simulink model "XSWIFT_cruise"  (R2025b)
settings: Solver=ode4  StartTime=0.0  StopTime=85  FixedStep=0.001  MaxStep=0.001  RelTol=1e-4
InitFcn:
  | [filepath, name] = fileparts(get_param(bdroot, 'FileName'))
  | if strcmp(filepath, pwd) ~= 1
  |     disp(strcat('cambiando el directorio actual a ', filepath))
  |     cd(filepath);
  | end
  | run(strcat(name, '_init'));
  | load("long_cruise.mat");
  | load("lat_cruise.mat")
values from neighbouring files (symbols this model uses):
  d2r = pi/180    (= 0.0174532925199)    [XSWIFT_cruise_init.m]
  data =     [XSWIFT_data.mat]
  init =     [XSWIFT_nav.mat]
  masa = data.mass.zfw + (data.mass.max_takeoff - data.mass.zfw) * mass_frac    [XSWIFT_cruise_init.m]
  nav =     [XSWIFT_nav.mat]
  obs_alpha_la = 20    [implementacion_digital_controles.m]    (also in long_cruise.mat)
  r = rad2deg(x(:,3))    [latero_direccional_LQR.m]
  r2d = 180/pi    (= 57.2957795131)    [XSWIFT_cruise_init.m]
  T_rec = 1/20    (= 0.05)    [XSWIFT_cruise_init.m]
  tau_filtro_lat = 0.3    [lat_cruise.mat]    (also in latero_direccional_LQR.m)
  Tc = 1/25    (= 0.04)    [XSWIFT_cruise_init.m]
  timeSince1970 = 1.3201e+09    (= 1320100000)    [XSWIFT_cruise_init.m]
  x_cg = 0    [XSWIFT_cruise_init.m]
  x_ref = 0    [XSWIFT_cruise_init.m]
undefined symbols (not defined in the file or in its folder): Earth, engine, F, m, MIL, Moderate, s, WGS84, wind
libraries: simulink x6, aerolibconvert2 x4, aerolibasang x4, aerolibfltsims x4, aerolibactuator x3, aerolibwind2 x2, aerolib6dof2 x1, aerolibadyn x1, aerolibatmos2 x1, aerolibanimutils x1, aerolibconvert x1, aerolibobsolete x1
(part 2 of 2)

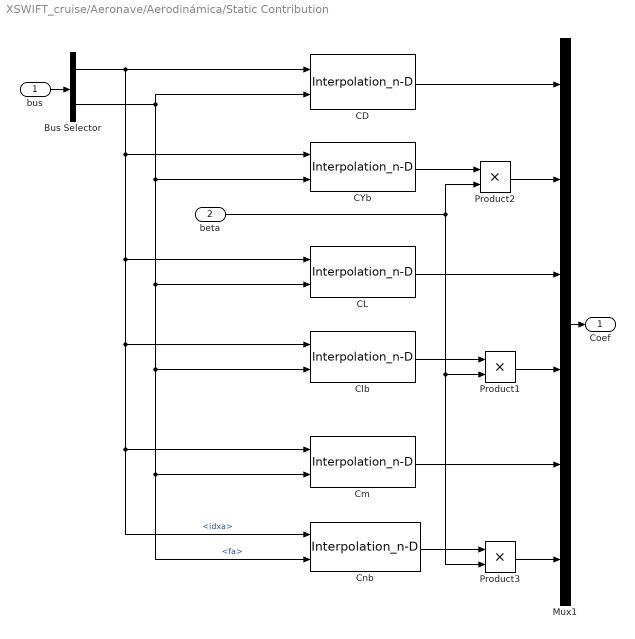
== system XSWIFT_cruise/Aeronave/Aerodinámica/Static Contribution ==
  bus : Inport
  beta : Inport  Port=2
  Bus Selector : BusSelector  OutputSignals=idxa,fa
  CD : Interpolation_n-D  NumberOfTableDimensions=1  Table="permute(data.cd,[1  2])"  OutDataTypeStr=double
      settings: InputPortMap=u0,u1
  CL : Interpolation_n-D  NumberOfTableDimensions=1  Table="permute(data.cl,[1  2])"  ExtrapMethod=Clip  OutDataTypeStr=double
      settings: InputPortMap=u0,u1
  CYb : Interpolation_n-D  NumberOfTableDimensions=1  Table="permute(data.cyb,[1  2])"  OutDataTypeStr=double
      settings: InputPortMap=u0,u1
  Clb : Interpolation_n-D  NumberOfTableDimensions=1  Table="permute(data.clb,[1  2])"  OutDataTypeStr=double
      settings: InputPortMap=u0,u1
  Cm : Interpolation_n-D  NumberOfTableDimensions=1  Table="permute(data.cm,[1  2])"  ExtrapMethod=Clip  OutDataTypeStr=double
      settings: InputPortMap=u0,u1
  Cnb : Interpolation_n-D  NumberOfTableDimensions=1  Table="permute(data.cnb,[1  2])"  OutDataTypeStr=double
      settings: InputPortMap=u0,u1
  Mux1 : Mux  Inputs=6
  Product1 : Product  RndMeth=Zero
  Product2 : Product  RndMeth=Zero
  Product3 : Product  RndMeth=Zero
  Coef : Outport
  wires:
  Bus Selector/1 -> CD/1, CYb/1, Clb/1, Cnb/1, Cm/1, CL/1  "<idxa>"
  Bus Selector/2 -> CD/2, CYb/2, Clb/2, Cnb/2, Cm/2, CL/2  "<fa>"
  CD/1 -> Mux1/1
  CL/1 -> Mux1/3
  CYb/1 -> Product2/1
  Clb/1 -> Product1/1
  Product2/1 -> Mux1/2
  Product1/1 -> Mux1/4
  Cm/1 -> Mux1/5
  Cnb/1 -> Product3/1
  beta/1 -> Product1/2, Product3/2, Product2/2
  Product3/1 -> Mux1/6
  Mux1/1 -> Coef/1
  bus/1 -> Bus Selector/1

== system XSWIFT_cruise/Aeronave/Flight Parameters/module ==
  vec : Inport
  Dot Product : DotProduct  OutDataTypeStr=Inherit: Inherit via internal rule
  Sqrt : Sqrt
  norm : Outport
  wires:
  vec/1 -> Dot Product/1, Dot Product/2
  Dot Product/1 -> Sqrt/1
  Sqrt/1 -> norm/1

== system XSWIFT_cruise/FCC/NAV/ned//enu ==
  x : Inport
  Gain : Gain  Gain=[1 1 -1]
  Selector4 : Selector  InputPortWidth=3  IndexOptions=Index vector (dialog)  Indices=[2 1 3]  OutputSizes=1
  y : Outport
  wires:
  x/1 -> Gain/1
  Selector4/1 -> y/1
  Gain/1 -> Selector4/1

== system XSWIFT_cruise/Aeronave/Aerodinámica/Control Contribution/Alerones ==
  idxa : Inport
  fa : Inport  Port=2
  delta : Inport  Port=3
  (delta aileron) : PreLookup  BreakpointsData=data.aler.delta  BeginIndexSearchUsingPreviousIndexResult=on  ExtrapMethod=Linear  IndexDataTypeStr=int32  FractionDataTypeStr=double
  Cl roll : Interpolation_n-D  NumberOfTableDimensions=1  Table=data.aler.clroll  OutDataTypeStr=double
      settings: InputPortMap=u0,u1
  Cn roll : Interpolation_n-D  Table=data.aler.cn  OutDataTypeStr=double
  Cn : Outport
  Cl : Outport  Port=2
  wires:
  (delta aileron)/1 -> Cl roll/1, Cn roll/3
  (delta aileron)/2 -> Cl roll/2, Cn roll/4
  idxa/1 -> Cn roll/1
  fa/1 -> Cn roll/2
  Cn roll/1 -> Cn/1
  delta/1 -> (delta aileron)/1
  Cl roll/1 -> Cl/1

== system XSWIFT_cruise/Aeronave/Aerodinámica/Control Contribution/Elevador ==
  idxa : Inport
  fa : Inport  Port=2
  delta : Inport  Port=3
  (delta elevator) : PreLookup  BreakpointsData=data.elev.delta  BeginIndexSearchUsingPreviousIndexResult=on  ExtrapMethod=Linear  IndexDataTypeStr=int32  FractionDataTypeStr=double
  D(CD) : Interpolation_n-D  NumberOfTableDimensions=1  Table=data.elev.dcdmin  ExtrapMethod=Clip  OutDataTypeStr=double
      settings: InputPortMap=u0,u1
  D(CDi) : Interpolation_n-D  Table=data.elev.dcdi  OutDataTypeStr=double
  D(CL) : Interpolation_n-D  NumberOfTableDimensions=1  Table=data.elev.dcl  OutDataTypeStr=double
      settings: InputPortMap=u0,u1
  D(Cm) : Interpolation_n-D  NumberOfTableDimensions=1  Table=data.elev.dcm  OutDataTypeStr=double
      settings: InputPortMap=u0,u1
  Sum : Sum  Inputs=|++
  CD : Outport
  CL : Outport  Port=2
  CM : Outport  Port=3
  wires:
  (delta elevator)/1 -> D(Cm)/1, D(CL)/1, D(CD)/2, D(CD)/1, D(CDi)/3
  (delta elevator)/2 -> D(CL)/2, D(Cm)/2, D(CDi)/4
  idxa/1 -> D(CDi)/1
  fa/1 -> D(CDi)/2
  delta/1 -> (delta elevator)/1
  D(CL)/1 -> CL/1
  D(Cm)/1 -> CM/1
  D(CDi)/1 -> Sum/1
  Sum/1 -> CD/1
  D(CD)/1 -> Sum/2

== system XSWIFT_cruise/Aeronave/Aerodinámica/Control Contribution/Rudder ==
  delta : Inport
  (delta timon) : PreLookup  BreakpointsData=data.rudr.delta  BeginIndexSearchUsingPreviousIndexResult=on  ExtrapMethod=Linear  IndexDataTypeStr=int32  FractionDataTypeStr=double
  D(CL) : Interpolation_n-D  NumberOfTableDimensions=1  Table=data.rudr.dcy  ExtrapMethod=Clip  OutDataTypeStr=double
      settings: InputPortMap=u0,u1
  D(CL)1 : Interpolation_n-D  NumberOfTableDimensions=1  Table=data.rudr.dcd  ExtrapMethod=Clip  OutDataTypeStr=double
      settings: InputPortMap=u0,u1
  D(Cn) : Interpolation_n-D  NumberOfTableDimensions=1  Table=data.rudr.dcn  ExtrapMethod=Clip  OutDataTypeStr=double
      settings: InputPortMap=u0,u1
  CD : Outport
  CN : Outport  Port=2
  Cn : Outport  Port=3
  wires:
  delta/1 -> (delta timon)/1
  (delta timon)/1 -> D(CL)1/1, D(CL)/1, D(Cn)/1
  (delta timon)/2 -> D(CL)1/2, D(CL)/2, D(Cn)/2
  D(CL)1/1 -> CD/1
  D(CL)/1 -> CN/1
  D(Cn)/1 -> Cn/1

== matlab function XSWIFT_cruise/FCC/MATLAB Function ==
  data: de output; beta input; da output; p input; r input; phi input; psi input; psi_ref input; V_real input; V_des input; alpha_meas input; q input; theta input; h input; h_ref input; dr output; Tcmd output
function [de, da, dr, Tcmd] = implementacion_digital_controles( ...
    beta, p, r, phi, psi, psi_ref, ...        % --- lateral
    V_real,V_des, alpha_meas, q, theta, h, h_ref)   % --- longitudinal
[de, da, dr, Tcmd] = implementacion_digital_controles( ...
    beta, p, r, phi, psi, psi_ref, ...        % --- lateral
    V_real,V_des,  alpha_meas, q, theta, h, h_ref)
end
